simulink model "sim_st_smc"  (R2023b)
settings: Solver=ode1  StartTime=0.0  StopTime=2  FixedStep=0.0001  RelTol=1e-3
values from neighbouring files (symbols this model uses):
  Te = 0.001    [ai_smc.m]    (also in fsmc.m; ismc.m; st_smc.m)
  Tm = 0.2    [ai_smc.m]    (also in fsmc.m; ismc.m; st_smc.m)
  ts = 1e-4    (= 0.0001)    [ai_smc.m]    (also in fsmc.m; ismc.m; st_smc.m)
settings Model: Creator=HP  LastModifiedBy=HP

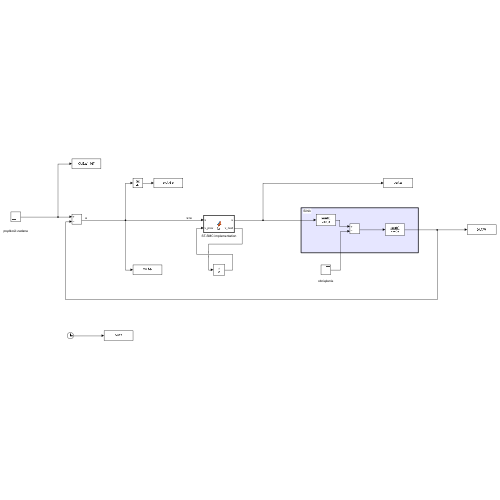
[thumbnail: Simulink's stored preview of the top-level diagram]
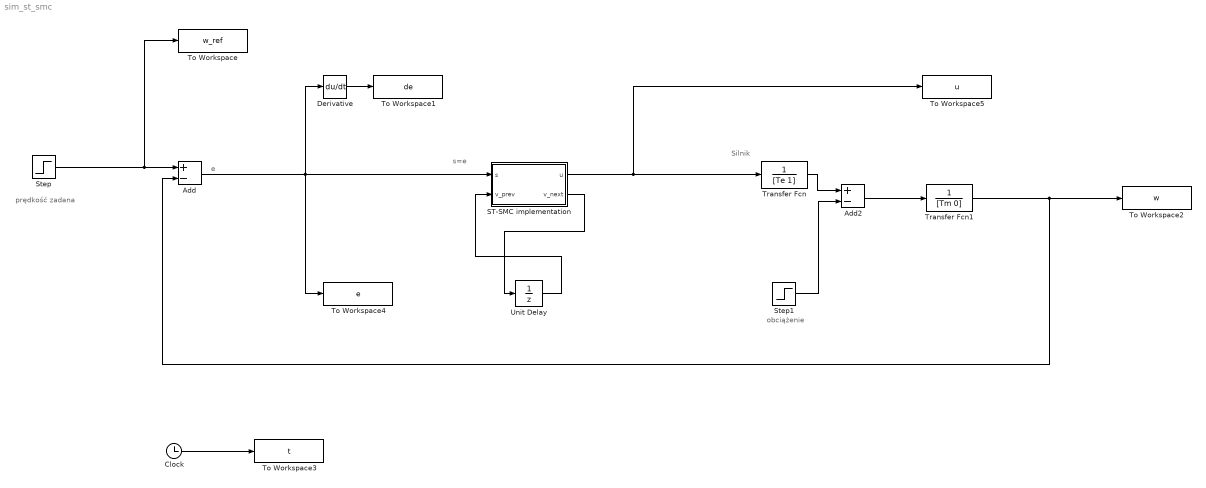
== system sim_st_smc ==
  note: s=e
  note: e
  note: Silnik
  note: prędkość zadana
  note: obciążenie
  Add : Sum  Inputs=+-
  Add2 : Sum  Inputs=+-
  Clock : Clock
  Derivative : Derivative
  ST-SMC implementation : MATLAB Function  TreatAsAtomicUnit=on
  Step : Step  Time=0.1  SampleTime=0
  Step1 : Step  SampleTime=0
  To Workspace : ToWorkspace  VariableName=w_ref  SaveFormat=Timeseries  SampleTime=-1
  To Workspace1 : ToWorkspace  VariableName=de  SaveFormat=Timeseries  SampleTime=-1
  To Workspace2 : ToWorkspace  VariableName=w  SaveFormat=Timeseries  SampleTime=-1
  To Workspace3 : ToWorkspace  VariableName=t  SaveFormat=Timeseries  SampleTime=-1
  To Workspace4 : ToWorkspace  VariableName=e  SaveFormat=Timeseries  SampleTime=-1
  To Workspace5 : ToWorkspace  VariableName=u  SaveFormat=Timeseries  SampleTime=-1
  Transfer Fcn : TransferFcn  Denominator=[Te 1]
  Transfer Fcn1 : TransferFcn  Denominator=[Tm 0]
  Unit Delay : UnitDelay  SampleTime=ts  HasFrameUpgradeWarning=on
  wires:
  Clock/1 -> To Workspace3/1
  Transfer Fcn1/1 -> To Workspace2/1, Add/2
  Step1/1 -> Add2/2
  Add2/1 -> Transfer Fcn1/1
  Transfer Fcn/1 -> Add2/1
  Derivative/1 -> To Workspace1/1
  Unit Delay/1 -> ST-SMC implementation/2(v_prev)
  Step/1 -> To Workspace/1, Add/1
  ST-SMC implementation/1(u) -> Transfer Fcn/1, To Workspace5/1
  ST-SMC implementation/2(v_next) -> Unit Delay/1
  Add/1 -> ST-SMC implementation/1(s), Derivative/1, To Workspace4/1

== matlab function sim_st_smc/ST-SMC implementation ==
  data: s input; u output; v_prev input; v_next output
function [u, v_next] = fcn(s, v_prev)
% Super-Twisting Sliding Mode Controller (ST-SMC) - implementacja dyskretna

% Wejścia:
%   s       – powierzchnia poślizgu (s = e + λ·de)
%   v_prev  – poprzednia wartość pomocniczej zmiennej v(k−1)
%
% Wyjścia:
%   u       – wyjściowy sygnał sterujący (ograniczony)
%   v_next  – zaktualizowana wartość zmiennej v(k)

ts = 1e-4;      % krok dyskretyzacji (zgodny z parametrem ts w MATLAB workspace)
k1 = 8;         % współczynnik wzmocnienia dla składnika pierwiastkowego (u1)
k2 = 1;         % współczynnik wzmocnienia dla składnika całkującego (u2)
eps = 1e-3;     % mała wartość zapobiegająca skokom sygnału w sign(s)
eps2 = 1e-12;   % minimalna wartość dodana do sqrt(), by uniknąć sqrt(0)
u_max = 10;     % maksymalna dopuszczalna wartość sterowania (ograniczenie nasycenia)

% -------------------------------------------------------------------------
% 1) Przybliżony operator sign(s)
% -------------------------------------------------------------------------
% Zamiast idealnego sign(s), który powoduje oscylacje (chattering),
% stosujemy wersję wygładzoną: s/eps ograniczoną do zakresu [-1, 1].
% Dla |s| < eps otrzymujemy przejście płynne przez zero.
sign_approx = max(-1, min(1, s/eps));

% -------------------------------------------------------------------------
% 2) Dyskretna integracja składowej v
% -------------------------------------------------------------------------
% Zmienna v jest pomocniczą składową całkującą w algorytmie Super-Twisting.
% Tu implementujemy całkowanie metodą Eulera w czasie dyskretnym.
v_next = v_prev + ts * sign_approx;

% -------------------------------------------------------------------------
% 3) Składowa pierwiastkowa (u1)
% -------------------------------------------------------------------------
% Pierwszy człon sterowania ST-SMC odpowiada za szybkie „ściąganie” stanu
% do powierzchni poślizgu. Zawiera pierwiastek z |s| i znak (sign).
% Uwaga: odwrócony znak wynika z przyjętej konwencji w modelu Simulinka.
u1 = k1 * sqrt(abs(s) + eps2) * sign_approx;

% -------------------------------------------------------------------------
% 4) Składowa zależna od v (u2)
% -------------------------------------------------------------------------
% Drugi człon sterowania stabilizuje układ po osiągnięciu powierzchni s=0.
% Wartość v_next pochodzi z kroku (2).
% Znak jest odwrócony (zgodnie z przyjętym modelem dynamicznym).
u2 = k2 * v_next;

% -------------------------------------------------------------------------
% 5) Suma obu składników i ograniczenie nasycenia
% -------------------------------------------------------------------------
% Ostateczne sterowanie jest sumą u1 i u2, ale ograniczamy je do ±u_max,
% aby zapobiec zbyt dużym wartościom sygnału wysyłanego do obiektu.
u_raw = u1 + u2;
u = max(-u_max, min(u_max, u_raw));   % saturacja sygnału sterującego

end
